simulink model "uDAQ28LT_system"  (R2020b)
settings: Solver=VariableStepAuto  StartTime=0.0  StopTime=t_sim  RelTol=1e-3
values from neighbouring files (symbols this model uses):
  in_bulb = 0    [uDAQ28LT_variables.mat]
  in_fan = 0    [uDAQ28LT_variables.mat]
  in_led = 0    [uDAQ28LT_variables.mat]
  Kc = 0    [uDAQ28LT_variables.mat]
  reg_output = 0    [uDAQ28LT_variables.mat]
  reg_signal = 0    [uDAQ28LT_variables.mat]
  reg_target = 0    [uDAQ28LT_variables.mat]
  Ti = 0    [uDAQ28LT_variables.mat]
  Ts = block.DialogPrm(3).Data    [uDAQ28LT_fun.m]    (also in uDAQ28LT_variables.mat = 1)
  U_max = 0    [uDAQ28LT_variables.mat]
  U_min = 0    [uDAQ28LT_variables.mat]
libraries: uDAQ28LT_lib x2
settings Model: Creator=dp  LastModifiedBy=udaq

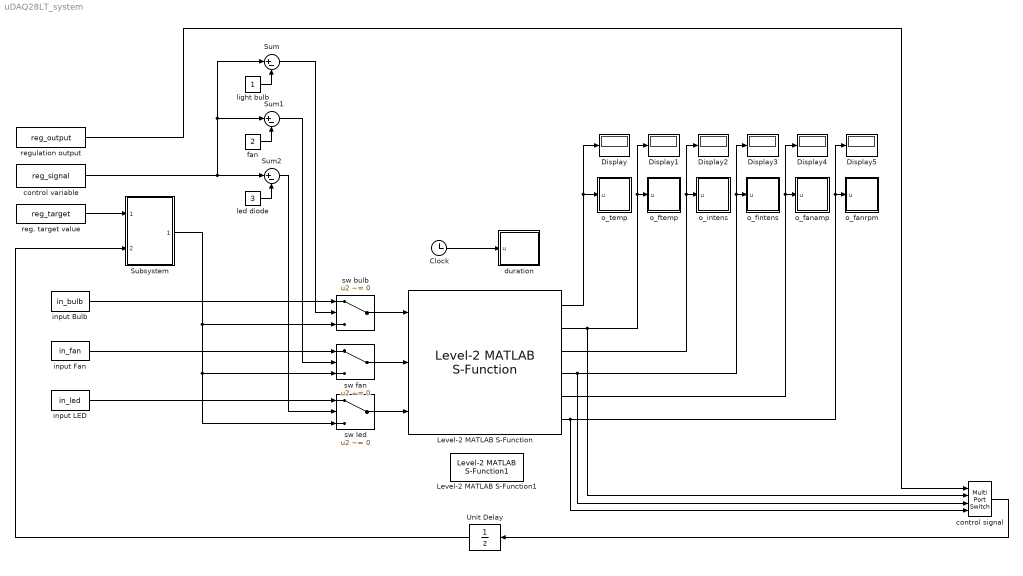
== system uDAQ28LT_system ==
  Clock : Clock
  Display{,1..5} (6 alike) : Display
  Level-2 MATLAB S-Function : uDAQ28LT_lib/Level-2 MATLAB S-Function  com=com  baud=baud  Ts=Ts
  Level-2 MATLAB S-Function1 : uDAQ28LT_lib/Level-2 MATLAB S-Function1  simTimePerRealTime=1
  Subsystem : Subsystem  mask{Kc=Kc, Ti=Ti, Umin=U_min, Umax=U_max}
      mask Display: disp('PI \nControl')
  Sum : Sum  Inputs=|+-
  Sum1 : Sum  Inputs=|+-
  Sum2 : Sum  Inputs=|+-
  Unit Delay : UnitDelay  SampleTime=-1  HasFrameUpgradeWarning=on
  control signal : MultiPortSwitch  OutDataTypeStr=double  SampleTime=Ts
  control variable : Constant  Value=reg_signal  SampleTime=Ts
  duration : MATLAB Function  TreatAsAtomicUnit=on  SystemSampleTime=Ts
  fan : Constant  Value=2  SampleTime=Ts
  input Bulb : Constant  Value=in_bulb  SampleTime=Ts
  input Fan : Constant  Value=in_fan  SampleTime=Ts
  input LED : Constant  Value=in_led  SampleTime=Ts
  led diode : Constant  Value=3  SampleTime=Ts
  light bulb : Constant  SampleTime=Ts
  o_fanamp : MATLAB Function  TreatAsAtomicUnit=on  SystemSampleTime=Ts
  o_fanrpm : MATLAB Function  TreatAsAtomicUnit=on  SystemSampleTime=Ts
  o_fintens : MATLAB Function  TreatAsAtomicUnit=on  SystemSampleTime=Ts
  o_ftemp : MATLAB Function  TreatAsAtomicUnit=on  SystemSampleTime=Ts
  o_intens : MATLAB Function  TreatAsAtomicUnit=on  SystemSampleTime=Ts
  o_temp : MATLAB Function  TreatAsAtomicUnit=on  SystemSampleTime=Ts
  reg. target value : Constant  Value=reg_target  SampleTime=Ts
  regulation output : Constant  Value=reg_output  SampleTime=Ts
  sw bulb : Switch  Criteria=u2 ~= 0  OutDataTypeStr=double
  sw fan : Switch  Criteria=u2 ~= 0  OutDataTypeStr=double
  sw led : Switch  Criteria=u2 ~= 0  OutDataTypeStr=double
  wires:
  Level-2 MATLAB S-Function/1 -> Display/1, o_temp/1(u)
  Level-2 MATLAB S-Function/2 -> Display1/1, o_ftemp/1(u), control signal/2
  Clock/1 -> duration/1(u)
  sw bulb/1 -> Level-2 MATLAB S-Function/1
  sw fan/1 -> Level-2 MATLAB S-Function/2
  sw led/1 -> Level-2 MATLAB S-Function/3
  light bulb/1 -> Sum/2
  fan/1 -> Sum1/2
  led diode/1 -> Sum2/2
  Level-2 MATLAB S-Function/3 -> Display2/1, o_intens/1(u)
  Level-2 MATLAB S-Function/4 -> Display3/1, o_fintens/1(u), control signal/3
  Level-2 MATLAB S-Function/5 -> Display4/1, o_fanamp/1(u)
  Level-2 MATLAB S-Function/6 -> Display5/1, o_fanrpm/1(u), control signal/4
  Sum/1 -> sw bulb/2
  Sum1/1 -> sw fan/2
  Sum2/1 -> sw led/2
  control variable/1 -> Sum/1, Sum1/1, Sum2/1
  input Bulb/1 -> sw bulb/1
  input Fan/1 -> sw fan/1
  input LED/1 -> sw led/1
  regulation output/1 -> control signal/1
  reg. target value/1 -> Subsystem/1(Required value)
  Subsystem/1(Control signal) -> sw bulb/3, sw led/3, sw fan/3
  control signal/1 -> Unit Delay/1
  Unit Delay/1 -> Subsystem/2(Output)

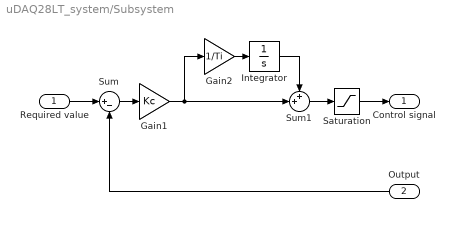
== system uDAQ28LT_system/Subsystem ==
  Required value : Inport
  Output : Inport  Port=2
  Gain1 : Gain  Gain=Kc
  Gain2 : Gain  Gain=1/Ti
  Integrator : Integrator
  Saturation : Saturate  UpperLimit=Umax  LowerLimit=Umin
  Sum : Sum  Inputs=|+-
  Sum1 : Sum  Inputs=++|
  Control signal : Outport
  wires:
  Saturation/1 -> Control signal/1
  Required value/1 -> Sum/1
  Sum/1 -> Gain1/1
  Output/1 -> Sum/2
  Gain1/1 -> Gain2/1, Sum1/2
  Sum1/1 -> Saturation/1
  Gain2/1 -> Integrator/1
  Integrator/1 -> Sum1/1

== matlab function uDAQ28LT_system/duration ==
  data: u input
function fcn(u)
%#codegen
coder.extrinsic('num2str');
coder.extrinsic('strcat');
coder.extrinsic('evalin');
evalin('base',strcat('duration(end+1)=', num2str(u),';'));
end

== matlab function uDAQ28LT_system/o_temp ==
  data: u input
function fcn(u)
%#codegen
coder.extrinsic('num2str');
coder.extrinsic('strcat');
coder.extrinsic('evalin');
evalin('base',strcat('o_temp(end+1)=', num2str(u),';'));
end

== matlab function uDAQ28LT_system/o_intens ==
  data: u input
function fcn(u)
%#codegen
coder.extrinsic('num2str');
coder.extrinsic('strcat');
coder.extrinsic('evalin');
evalin('base',strcat('o_intens(end+1)=', num2str(u),';'));
end

== matlab function uDAQ28LT_system/o_fintens ==
  data: u input
function fcn(u)
%#codegen
coder.extrinsic('num2str');
coder.extrinsic('strcat');
coder.extrinsic('evalin');
evalin('base',strcat('o_fintens(end+1)=', num2str(u),';'));
end

== matlab function uDAQ28LT_system/o_fanamp ==
  data: u input
function fcn(u)
%#codegen
coder.extrinsic('num2str');
coder.extrinsic('strcat');
coder.extrinsic('evalin');
evalin('base',strcat('o_fanamp(end+1)=', num2str(u),';'));
end

== matlab function uDAQ28LT_system/o_fanrpm ==
  data: u input
function fcn(u)
%#codegen
coder.extrinsic('num2str');
coder.extrinsic('strcat');
coder.extrinsic('evalin');
evalin('base',strcat('o_fanrpm(end+1)=', num2str(u),';'));
end

== matlab function uDAQ28LT_system/o_ftemp ==
  data: u input
function fcn(u)
%#codegen
coder.extrinsic('num2str');
coder.extrinsic('strcat');
coder.extrinsic('evalin');
evalin('base',strcat('o_ftemp(end+1)=', num2str(u),';'));
end
